simulink model "test_s_function"  (R2024a)
settings: Solver=VariableStepAuto  StartTime=0.0  StopTime=10.0  RelTol=1e-3
settings Model: Creator=sdcnlab  LastModifiedBy=sdcnlab

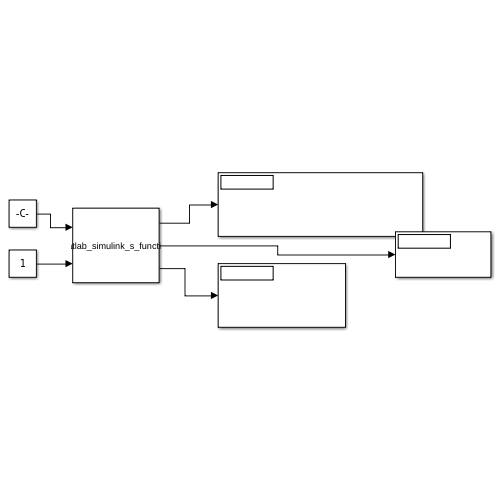
[thumbnail: Simulink's stored preview of the top-level diagram]
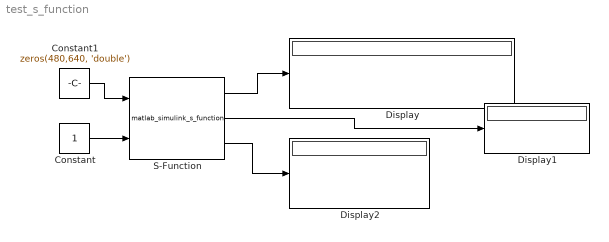
== system test_s_function ==
  Constant : Constant
  Constant1 : Constant  Value=zeros(480,640, 'double')
  Display : Display
  Display1 : Display
  Display2 : Display
  S-Function : S-Function  FunctionName=matlab_simulink_s_function  Parameters=2e-3,1280,1280,1,480,640  SFunctionDeploymentMode=off  EnableBusSupport=off
  wires:
  Constant/1 -> S-Function/2
  Constant1/1 -> S-Function/1
  S-Function/1 -> Display/1
  S-Function/3 -> Display2/1
  S-Function/2 -> Display1/1
